simulink model "a6222_b1"  (R2019a)
settings: Solver=VariableStepAuto  StartTime=0.0  StopTime=200  RelTol=1e-3
libraries: simulink x1
settings Model: Creator=Administrator  LastModifiedBy=Administrator

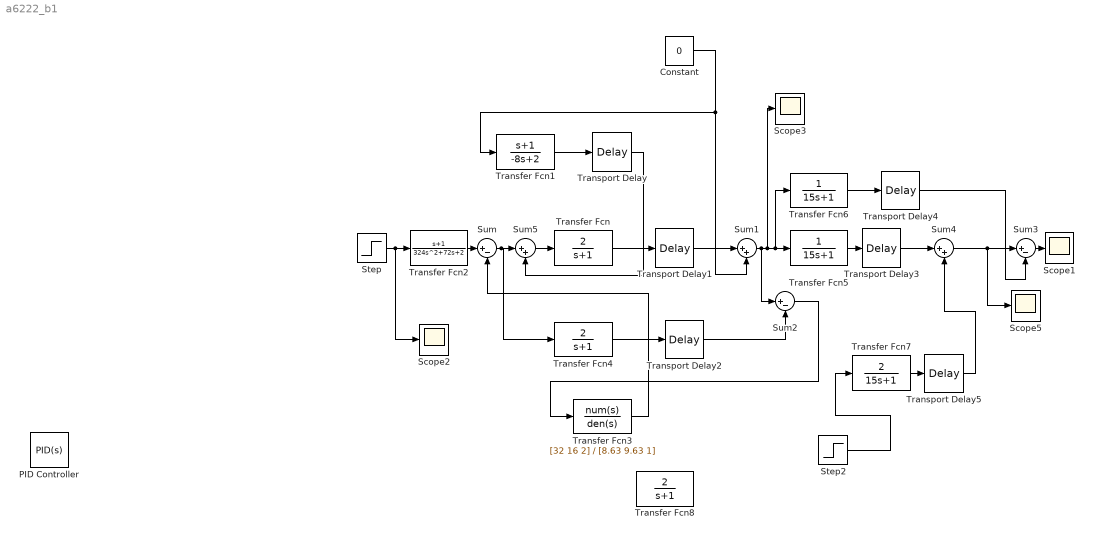
== system a6222_b1 ==
  Constant : Constant  Value=0
  PID Controller : simulink/Continuous/PID Controller  Controller=PID  Form=Parallel  TimeDomain=Continuous-time  SampleTime=-1  IntegratorMethod=Forward Euler  FilterMethod=Forward Euler  ControllerParametersSource=internal  P=11/3  I=1/3  D=10/3  UseFilter=on  N=100  TunerSelectOption=Transfer Function Based (PID Tuner App)  InitialConditionSource=internal  InitialConditionForIntegrator=0  InitialConditionForFilter=0  DifferentiatorICPrevScaledInput=0  ExternalReset=none  TrackingMode=off  Kt=1  LimitOutput=off  UpperSaturationLimit=inf  LowerSaturationLimit=-inf  LinearizeAsGain=on  AntiWindupMode=none  Kb=1  POutMin=[]  POutMax=[]  IOutMin=[]  IOutMax=[]  DOutMin=[]  DOutMax=[]  NOutMin=[]  NOutMax=[]  SumOutMin=[]  SumOutMax=[]  SaturationOutMin=[]  SaturationOutMax=[]  PParamMin=[]  PParamMax=[]  IParamMin=[]  IParamMax=[]  DParamMin=[]  DParamMax=[]  NParamMin=[]  NParamMax=[]  KbParamMin=[]  KbParamMax=[]  KtParamMin=[]  KtParamMax=[]  KbOutMin=[]  KbOutMax=[]  KtOutMin=[]  KtOutMax=[]  IntegratorOutMin=[]  IntegratorOutMax=[]  FilterOutMin=[]  FilterOutMax=[]  SumI1OutMin=[]  SumI1OutMax=[]  SumI2OutMin=[]  SumI2OutMax=[]  SumI3OutMin=[]  SumI3OutMax=[]  SumI4OutMin=[]  SumI4OutMax=[]  SumDOutMin=[]  SumDOutMax=[]  DifferentiatorOutMin=[]  DifferentiatorOutMax=[]  FilterDiffOutCoefMin=[]  FilterDiffOutCoefMax=[]  ReciprocalOutMin=[]  ReciprocalOutMax=[]  SumDenOutMin=[]  SumDenOutMax=[]  SumNumOutMin=[]  SumNumOutMax=[]  DivideOutMin=[]  DivideOutMax=[]  IntegratorContinuousStateAttributes=''  IntegratorStateMustResolveToSignalObject=off  IntegratorRTWStateStorageClass=Auto  FilterContinuousStateAttributes=''  FilterStateMustResolveToSignalObject=off  FilterRTWStateStorageClass=Auto  ParallelPVariant=InternalParameters  IdealPVariant=Disabled  IVariant=InternalParameters  DVariant=InternalParameters  IntegratorVariant=Continuous  SatVariant=Disabled  AWVariant=Passthrough  PCopyVariant=Disabled  TRVariant=Disabled  FdbkBlocksVariant=Forward  IdealPFdbkVariant=Disabled  SatFdbkVariant=Disabled  DerivativeFilterVariant=ContFilter  NVariant=InternalParameters  NCopyVariant=Disabled  FilterICVariant=InternalICsFilter  IntegratorICVariant=InternalICs  ExternalResetVariant=Disabled  TRSumVariant=Passthrough  SumFdbkVariant=Disabled  SumVariant=Sum_PID
  Scope{1..3,5} (4 alike) : Scope
  Step : Step  SampleTime=0
  Step2 : Step  Time=40  SampleTime=0
  Sum : Sum  Inputs=|+-
  Sum1 : Sum  Inputs=|++
  Sum2 : Sum  Inputs=|+-
  Sum3 : Sum  Inputs=|+-
  Sum4 : Sum  Inputs=|++
  Sum5 : Sum  Inputs=|++
  Transfer Fcn : TransferFcn  Numerator=[2]  Denominator=[1 1]
  Transfer Fcn1 : TransferFcn  Numerator=[1 1]  Denominator=[-8 2]
  Transfer Fcn2 : TransferFcn  Numerator=[1 1]  Denominator=[324 72 2]
  Transfer Fcn3 : TransferFcn  Numerator=[32 16 2]  Denominator=[8.63 9.63 1]
  Transfer Fcn4 : TransferFcn  Numerator=[2]  Denominator=[1 1]
  Transfer Fcn5 : TransferFcn  Denominator=[15 1]
  Transfer Fcn6 : TransferFcn  Denominator=[15 1]
  Transfer Fcn7 : TransferFcn  Numerator=[2]  Denominator=[15 1]
  Transfer Fcn8 : TransferFcn  Numerator=[2]  Denominator=[1 1]
  Transport Delay : TransportDelay  DelayTime=2
  Transport Delay1 : TransportDelay  DelayTime=4
  Transport Delay2 : TransportDelay  DelayTime=4
  Transport Delay3 : TransportDelay  DelayTime=20
  Transport Delay4 : TransportDelay  DelayTime=20
  Transport Delay5 : TransportDelay  DelayTime=30
  wires:
  Transfer Fcn1/1 -> Transport Delay/1
  Transfer Fcn/1 -> Transport Delay1/1
  Transport Delay1/1 -> Sum1/1
  Sum1/1 -> Scope3/1, Transfer Fcn6/1, Transfer Fcn5/1, Sum2/1
  Transfer Fcn4/1 -> Transport Delay2/1
  Sum/1 -> Transfer Fcn4/1, Sum5/1
  Transport Delay2/1 -> Sum2/2
  Step/1 -> Transfer Fcn2/1, Scope2/1
  Transfer Fcn2/1 -> Sum/1
  Sum2/1 -> Transfer Fcn3/1
  Transfer Fcn3/1 -> Sum/2
  Transfer Fcn5/1 -> Transport Delay3/1
  Transfer Fcn6/1 -> Transport Delay4/1
  Transport Delay4/1 -> Sum3/2
  Sum3/1 -> Scope1/1
  Step2/1 -> Transfer Fcn7/1
  Transfer Fcn7/1 -> Transport Delay5/1
  Transport Delay3/1 -> Sum4/1
  Sum4/1 -> Scope5/1, Sum3/1
  Transport Delay5/1 -> Sum4/2
  Constant/1 -> Transfer Fcn1/1, Sum1/2
  Sum5/1 -> Transfer Fcn/1
  Transport Delay/1 -> Sum5/2
